simulink subsystem "CiMappedEngine"  (R2025b)
settings: Solver=VariableStepAuto  StartTime=0.0  StopTime=10.0  RelTol=1e-3
undefined symbols (not defined in the file): Afr, BSFC, Ect, EgrVlvAreaPct, EngSpdOut, EngTrq, ExhCamPhase, ExhManGasTemp, FuelFlw, FuelVolFlw, IntkCamPhase, IntkPortFlw, IntkSwirlVlvPos, IntkVlvLift, NormAirChrg, PlntEngAccPwrTbl, PlntEngAccSpdBpt, PlntEngSinj, PlntEngTimeCECP, PlntEngTimeCEGR, PlntEngTimeCETC, PlntEngTimeCICP, PlntEngTimeCIRL, PlntEngTimeCIVL, PlntEngTimeCVCR, PlntEngTimeCVGT, PlntEngTimeCWGA, PlntEngTimeCWVA, ThrPosPct, TPCO, TPCO2, TPHC, TPNOx, TurboRackPos, VarCompRatioPos, VarIntkRunLen, WgAreaPct
libraries: autolibpowerinfoutils x1, autolibsharedmappedengines x1
(part 2 of 2)

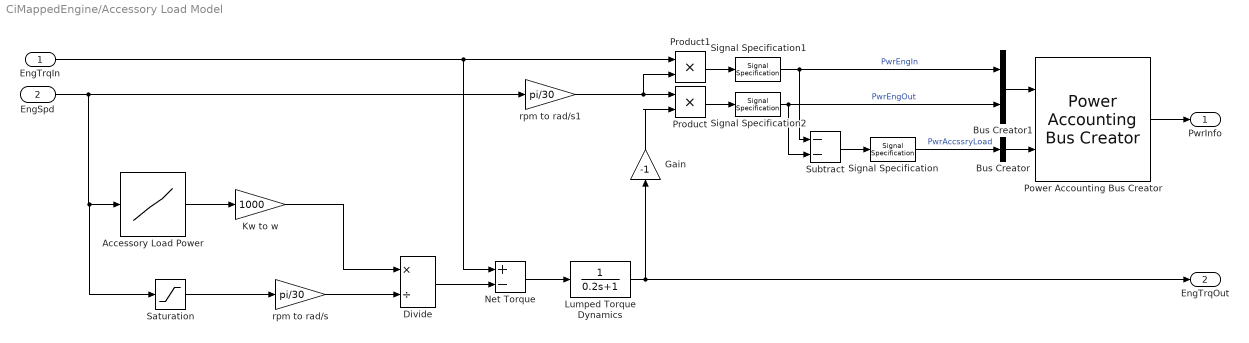
== system CiMappedEngine/Accessory Load Model ==
  EngTrqIn : Inport
  EngSpd : Inport  Port=2
  Accessory Load Power : Lookup_n-D  NumberOfTableDimensions=1  LookupTableObject=''  BreakpointsForDimension1=PlntEngAccSpdBpt  Table=PlntEngAccPwrTbl  ExtrapMethod=Clip  InternalRulePriority=Speed  RndMeth=Simplest
  Bus Creator : BusCreator  Inputs=1
  Bus Creator1 : BusCreator  Inputs=2
  Divide : Product  Inputs=*/
  Gain : Gain  Gain=-1
  Kw to w : Gain  Gain=1000
  Lumped Torque Dynamics : TransferFcn  Denominator=[0.2 1]
  Net Torque : Sum  Inputs=+-
  Power Accounting Bus Creator : autolibpowerinfoutils/Power Accounting Bus Creator  AssctBlkSelPopup=Parent  RefBlkName='libraryname/blkname'  PwrTrnsfrdCheckBox=on  PwrNotTrnsfrdCheckBox=on  PwrStoredCheckBox=off  aMode=6
  Product : Product
  Product1 : Product
  Saturation : Saturate  UpperLimit=Inf  LowerLimit=300
  Signal Specification : SignalSpecification  Unit=W
  Signal Specification1 : SignalSpecification  Unit=W
  Signal Specification2 : SignalSpecification  Unit=W
  Subtract : Sum  Inputs=--
  rpm to rad/s : Gain  Gain=pi/30
  rpm to rad/s1 : Gain  Gain=pi/30
  PwrInfo : Outport  VectorParamsAs1DForOutWhenUnconnected=off
  EngTrqOut : Outport  Port=2  Unit=N*m  VectorParamsAs1DForOutWhenUnconnected=off
  wires:
  Gain/1 -> Product/2
  Signal Specification2/1 -> Bus Creator1/2, Subtract/2  "PwrEngOut"
  Signal Specification1/1 -> Bus Creator1/1, Subtract/1  "PwrEngIn"
  rpm to rad/s1/1 -> Product/1, Product1/2
  Product1/1 -> Signal Specification1/1
  Product/1 -> Signal Specification2/1
  Power Accounting Bus Creator/1 -> PwrInfo/1
  Signal Specification/1 -> Bus Creator/1  "PwrAccssryLoad"
  Subtract/1 -> Signal Specification/1
  EngTrqIn/1 -> Net Torque/1, Product1/1
  Bus Creator1/1 -> Power Accounting Bus Creator/1
  Kw to w/1 -> Divide/1
  Bus Creator/1 -> Power Accounting Bus Creator/2
  Net Torque/1 -> Lumped Torque Dynamics/1
  Lumped Torque Dynamics/1 -> Gain/1, EngTrqOut/1
  rpm to rad/s/1 -> Divide/2
  Saturation/1 -> rpm to rad/s/1
  EngSpd/1 -> rpm to rad/s1/1, Accessory Load Power/1, Saturation/1
  Accessory Load Power/1 -> Kw to w/1
  Divide/1 -> Net Torque/2

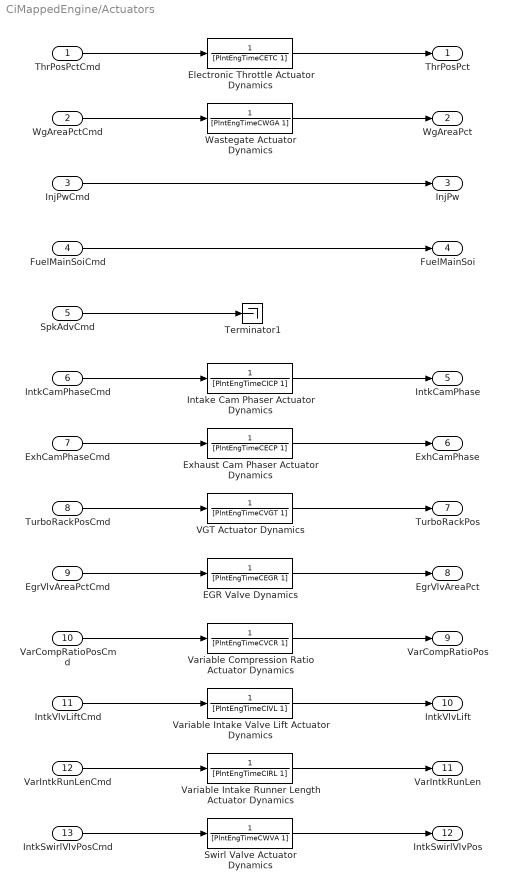
== system CiMappedEngine/Actuators ==
  ThrPosPctCmd : Inport  Unit=%
  WgAreaPctCmd : Inport  Port=2  Unit=%
  InjPwCmd : Inport  Port=3  Unit=ms
  FuelMainSoiCmd : Inport  Port=4  Unit=deg
  SpkAdvCmd : Inport  Port=5  Unit=deg
  IntkCamPhaseCmd : Inport  Port=6  Unit=deg
  ExhCamPhaseCmd : Inport  Port=7  Unit=deg
  TurboRackPosCmd : Inport  Port=8  Unit=1
  EgrVlvAreaPctCmd : Inport  Port=9  Unit=%
  VarCompRatioPosCmd : Inport  Port=10
  IntkVlvLiftCmd : Inport  Port=11
  VarIntkRunLenCmd : Inport  Port=12
  IntkSwirlVlvPosCmd : Inport  Port=13
  EGR Valve Dynamics : TransferFcn  Denominator=[PlntEngTimeCEGR 1]
  Electronic Throttle Actuator Dynamics : TransferFcn  Denominator=[PlntEngTimeCETC 1]
  Exhaust Cam Phaser Actuator Dynamics : TransferFcn  Denominator=[PlntEngTimeCECP 1]
  Intake Cam Phaser Actuator Dynamics : TransferFcn  Denominator=[PlntEngTimeCICP 1]
  Swirl Valve Actuator Dynamics : TransferFcn  Denominator=[PlntEngTimeCWVA 1]
  Terminator1 : Terminator
  VGT Actuator Dynamics : TransferFcn  Denominator=[PlntEngTimeCVGT 1]
  Variable Compression Ratio Actuator Dynamics : TransferFcn  Denominator=[PlntEngTimeCVCR 1]
  Variable Intake Runner Length Actuator Dynamics : TransferFcn  Denominator=[PlntEngTimeCIRL 1]
  Variable Intake Valve Lift Actuator Dynamics : TransferFcn  Denominator=[PlntEngTimeCIVL 1]
  Wastegate Actuator Dynamics : TransferFcn  Denominator=[PlntEngTimeCWGA 1]
  ThrPosPct : Outport  Unit=%  VectorParamsAs1DForOutWhenUnconnected=off
  WgAreaPct : Outport  Port=2  Unit=%  VectorParamsAs1DForOutWhenUnconnected=off
  InjPw : Outport  Port=3  VectorParamsAs1DForOutWhenUnconnected=off
  FuelMainSoi : Outport  Port=4  VectorParamsAs1DForOutWhenUnconnected=off
  IntkCamPhase : Outport  Port=5  Unit=deg  VectorParamsAs1DForOutWhenUnconnected=off
  ExhCamPhase : Outport  Port=6  Unit=deg  VectorParamsAs1DForOutWhenUnconnected=off
  TurboRackPos : Outport  Port=7  Unit=1  VectorParamsAs1DForOutWhenUnconnected=off
  EgrVlvAreaPct : Outport  Port=8  Unit=%  VectorParamsAs1DForOutWhenUnconnected=off
  VarCompRatioPos : Outport  Port=9  VectorParamsAs1DForOutWhenUnconnected=off
  IntkVlvLift : Outport  Port=10  VectorParamsAs1DForOutWhenUnconnected=off
  VarIntkRunLen : Outport  Port=11  VectorParamsAs1DForOutWhenUnconnected=off
  IntkSwirlVlvPos : Outport  Port=12  VectorParamsAs1DForOutWhenUnconnected=off
  wires:
  Variable Compression Ratio Actuator Dynamics/1 -> VarCompRatioPos/1
  Variable Intake Valve Lift Actuator Dynamics/1 -> IntkVlvLift/1
  Variable Intake Runner Length Actuator Dynamics/1 -> VarIntkRunLen/1
  Swirl Valve Actuator Dynamics/1 -> IntkSwirlVlvPos/1
  Intake Cam Phaser Actuator Dynamics/1 -> IntkCamPhase/1
  Exhaust Cam Phaser Actuator Dynamics/1 -> ExhCamPhase/1
  Wastegate Actuator Dynamics/1 -> WgAreaPct/1
  Electronic Throttle Actuator Dynamics/1 -> ThrPosPct/1
  FuelMainSoiCmd/1 -> FuelMainSoi/1
  IntkVlvLiftCmd/1 -> Variable Intake Valve Lift Actuator Dynamics/1
  IntkSwirlVlvPosCmd/1 -> Swirl Valve Actuator Dynamics/1
  WgAreaPctCmd/1 -> Wastegate Actuator Dynamics/1
  ThrPosPctCmd/1 -> Electronic Throttle Actuator Dynamics/1
  ExhCamPhaseCmd/1 -> Exhaust Cam Phaser Actuator Dynamics/1
  IntkCamPhaseCmd/1 -> Intake Cam Phaser Actuator Dynamics/1
  VarCompRatioPosCmd/1 -> Variable Compression Ratio Actuator Dynamics/1
  VarIntkRunLenCmd/1 -> Variable Intake Runner Length Actuator Dynamics/1
  InjPwCmd/1 -> InjPw/1
  VGT Actuator Dynamics/1 -> TurboRackPos/1
  EGR Valve Dynamics/1 -> EgrVlvAreaPct/1
  TurboRackPosCmd/1 -> VGT Actuator Dynamics/1
  EgrVlvAreaPctCmd/1 -> EGR Valve Dynamics/1
  SpkAdvCmd/1 -> Terminator1/1
